simulink model "Reading_Project_model"  (R2019a)
settings: Solver=VariableStepAuto  StartTime=0.0  StopTime=500  MaxStep=0.01  RelTol=1e-3
model workspace: external: MAT-File C:\Kisisel\MATLAB_Workspace\CMP684\NeuralNetworkProject\Lu2018_retry\Lu2018_ws.mat (data not in the file)
values from neighbouring files (symbols this model uses):
  chi = 25    [Reading_Project.mat]    (also in Reading_Project_script.m)
  coupling_matrix = [6.45637  1.27814  2.15629; -1.25619  0.91756  -1.67264; 1.11687  2.48901  -0.83674; 1.23637  -2.6581  -1.12503]    [Reading_Project.mat]    (also in Reading_Project_script.m = [     6.45637     1.27814     2.15629)
  Delta_J = [0  0  0; 0  0  0; 0  0  0]    [Reading_Project.mat]    (also in Reading_Project_script.m = diag([0 0 0]'))
  epsilon = 0.1    [Reading_Project.mat]    (also in Reading_Project_script.m)
  eta_init = [0.01242 0.01584 -0.01749 0.01125]    [Reading_Project.mat]    (also in Reading_Project_script.m = [0.01242, 0.01584, -0.01749, 0.01125]')
  gamma = 0.35    [Reading_Project.mat]    (also in Reading_Project_script.m)
  iota1 = 3    [Reading_Project.mat]    (also in Reading_Project_script.m)
  iota2 = 5    [Reading_Project.mat]    (also in Reading_Project_script.m)
  J = [800.027  0  0; 0  839.93  0; 0  0  289.93]    [Reading_Project.mat]    (also in Reading_Project_script.m = J0 + Delta_J)
  J0 = [800.027  0  0; 0  839.93  0; 0  0  289.93]    [Reading_Project.mat]    (also in Reading_Project_script.m = [  800.027   0           0)
  K = [1.20406729 0 0 0 0 1.62843121 0 0 0 0 2.73505444 0 ... (16 elements, 4x4)]    [Reading_Project.mat]    (also in Reading_Project_script.m = diag(omega_n.^2))
  K1 = [0.5  0  0; 0  0.5  0; 0  0  0.5]    [Reading_Project.mat]    (also in Reading_Project_script.m = diag(k1))
  k1 = [0.5 0.5 0.5]    [Reading_Project.mat]    (also in Reading_Project_script.m = [k11, k12, k13]')
  K2 = [0.5  0  0; 0  0.5  0; 0  0  0.5]    [Reading_Project.mat]    (also in Reading_Project_script.m = diag(k2))
  k2 = [0.5 0.5 0.5]    [Reading_Project.mat]    (also in Reading_Project_script.m = [k21, k22, k23]')
  L = [0.10973 0 0 0 0 0.153132 0 0 0 0 0.264608 0 ... (16 elements, 4x4)]    [Reading_Project.mat]    (also in Reading_Project_script.m = diag(2*omega_n.*zeta))
  lambda = 0.6    [Reading_Project.mat]    (also in Reading_Project_script.m)
  omega_init = [0 0 0]    [Reading_Project.mat]    (also in Reading_Project_script.m = [0, 0, 0]')
  q_init = [0.3 -0.2 -0.3 0.8832]    [Reading_Project.mat]    (also in Reading_Project_script.m = [0.3, -0.2, -0.3, 0.8832]')
  q_p = 0.6    [Reading_Project.mat]    (also in Reading_Project_script.m)
  qd_init = [0 0 0 1]    [Reading_Project.mat]    (also in Reading_Project_script.m = [0, 0, 0, 1]')
  sigma1 = 100    [Reading_Project.mat]    (also in Reading_Project_script.m)
  sigma2 = 0.01    [Reading_Project.mat]    (also in Reading_Project_script.m)
  tau = 10    [Reading_Project.mat]    (also in Reading_Project_script.m)
  um = 68    [Reading_Project.mat]    (also in Reading_Project_script.m)
  weight_init = [0.814723686393 0.905791937076 0.126986816294 0.913375856139 0.632359246225 0.0975404049994 0.278498218867 0.546881519205 0.957506835434 0.964888535199 0.157613081678 0.970592781761 ... (75 elements, 3x25)]    [Reading_Project.mat]    (also in Reading_Project_script.m = rand(3,25))
settings Model: Creator=kocab  LastModifiedBy=kocab

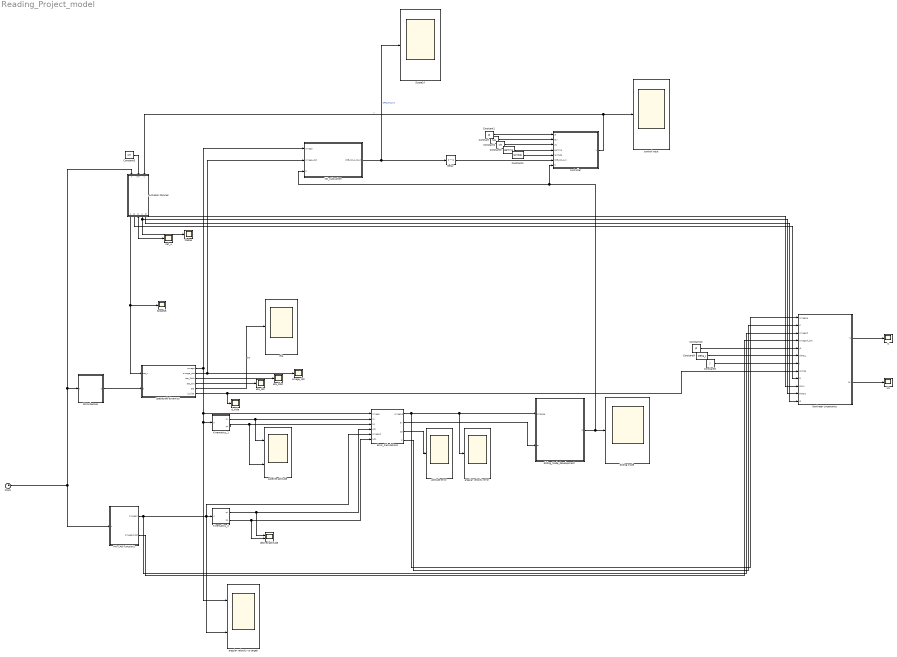
== system Reading_Project_model ==
  Actuator Failures : MATLAB Function  TreatAsAtomicUnit=on
  Clock : Clock
  Constant : Constant  Value=tau
  Constant1 : Constant  Value=J0
  Constant10 : Constant  Value=J0
  Constant2 : Constant  Value=chi
  Constant3 : Constant  Value=gamma
  Constant4 : Constant  Value=lambda
  Constant5 : Constant  Value=um
  Constant8 : Constant  Value=J
  Constant9 : Constant  Value=Delta_J
  Delay : Delay  DelayLength=1  InitialCondition=zeros(3,1)
  Disturbances : MATLAB Function  TreatAsAtomicUnit=on
  Error_Calculations : Subsystem
  Kinematics_1 : Subsystem
  Kinematics_2 : Subsystem
  MATLAB Function1 : MATLAB Function  TreatAsAtomicUnit=on
  N : Scope
  N1 : Scope
  NN_subsystem : Subsystem
  Nonlinear Uncertainty : MATLAB Function  TreatAsAtomicUnit=on
  Scope14 : Scope
  Scope15 : Scope
  Sliding mode : Scope
  Sliding_Mode_Development : Subsystem
  Spacecraft dynamics : Subsystem
  angular velocity error : Scope
  angular velocity vs target : Scope  NumInputPorts=2
  attitude error : Scope
  control input : Scope
  controller : MATLAB Function  TreatAsAtomicUnit=on
  d_tilda : Scope
  desired attitude : Scope  NumInputPorts=2
  eta : Scope
  eta_2dot : Scope
  eta_dot : Scope
  omega_dot : Scope
  sat_u : Scope
  satellite attitude : Scope  NumInputPorts=2
  thetao : Scope
  wires:
  Spacecraft dynamics/1(omega) -> angular velocity vs target/1, Kinematics_1/1(w), Error_Calculations/1(omega), NN_subsystem/1(omega)
  Spacecraft dynamics/5(eta) -> eta/1  "eta"
  Spacecraft dynamics/4(eta_dot) -> eta_dot/1
  Spacecraft dynamics/3(eta_2dot) -> eta_2dot/1
  Spacecraft dynamics/2(omega_dot) -> NN_subsystem/2(omega_dot), omega_dot/1
  MATLAB Function1/1(omegad) -> angular velocity vs target/2, Kinematics_2/1(w), Error_Calculations/5(omegad), Nonlinear Uncertainty/3(omegad)
  Clock/1 -> Actuator Failures/1(t), Disturbances/1(t), MATLAB Function1/1(t)
  Kinematics_1/1(qv) -> satellite attitude/1, Error_Calculations/2(qv)
  Kinematics_1/2(q4) -> satellite attitude/2, Error_Calculations/3(q4)
  Kinematics_2/2(q4) -> desired attitude/2, Error_Calculations/6(qd4)
  Kinematics_2/1(qv) -> Error_Calculations/4(qdv), desired attitude/1
  Disturbances/1(d) -> Spacecraft dynamics/2(d)
  Sliding_Mode_Development/1(S) -> NN_subsystem/3(S), controller/7(S), Sliding mode/1
  NN_subsystem/1(CPB_NN_output) -> Scope14/1, Delay/1  "CPB_NN_out"
  Constant/1 -> controller/2(tau)
  Constant1/1 -> controller/1(J0)
  Constant2/1 -> controller/3(chi)
  Constant3/1 -> controller/4(gamma)
  Constant4/1 -> controller/5(lambda)
  Error_Calculations/1(omegae) -> angular velocity error/1, Sliding_Mode_Development/1(omegae), Nonlinear Uncertainty/1(omegae)
  Error_Calculations/2(ev) -> Sliding_Mode_Development/2(ev)
  Error_Calculations/3(qe) -> attitude error/1
  Actuator Failures/4(thetao) -> thetao/1, Nonlinear Uncertainty/11(thetao)
  Actuator Failures/2(D) -> Nonlinear Uncertainty/9(D)
  Constant8/1 -> Nonlinear Uncertainty/7(J)
  Constant9/1 -> Nonlinear Uncertainty/6(delta_J)
  Constant10/1 -> Nonlinear Uncertainty/5(J0)
  Error_Calculations/4(C) -> Nonlinear Uncertainty/2(C)
  MATLAB Function1/2(omegad_dot) -> Nonlinear Uncertainty/4(omegad_dot)
  Spacecraft dynamics/6(d_tilda) -> Nonlinear Uncertainty/8(d_tilda), d_tilda/1
  Nonlinear Uncertainty/1(N) -> N/1
  controller/1(u) -> Actuator Failures/3(u), control input/1  "u"
  Delay/1 -> controller/6(CPB_NN_out)
  Nonlinear Uncertainty/2(N1) -> N1/1
  Actuator Failures/1(real_torque) -> Scope15/1, Spacecraft dynamics/1(sat_u)
  Constant5/1 -> Actuator Failures/2(um)
  Actuator Failures/3(sat_u) -> sat_u/1, Nonlinear Uncertainty/10(sat_u)
  Actuator Failures/5(G) -> Nonlinear Uncertainty/12(G)

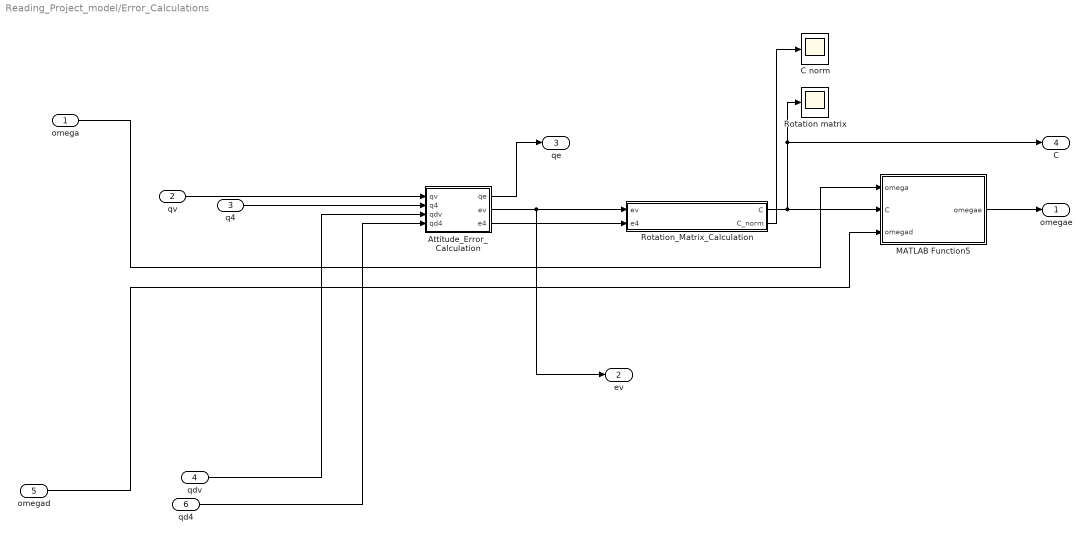
== system Reading_Project_model/Error_Calculations ==
  omega : Inport
  qv : Inport  Port=2
  q4 : Inport  Port=3
  qdv : Inport  Port=4
  omegad : Inport  Port=5
  qd4 : Inport  Port=6
  Attitude_Error_Calculation : MATLAB Function  TreatAsAtomicUnit=on
  C norm : Scope
  MATLAB Function5 : MATLAB Function  TreatAsAtomicUnit=on
  Rotation matrix : Scope
  Rotation_Matrix_Calculation : MATLAB Function  TreatAsAtomicUnit=on
  omegae : Outport
  ev : Outport  Port=2
  qe : Outport  Port=3
  C : Outport  Port=4
  wires:
  q4/1 -> Attitude_Error_Calculation/2(q4)
  Rotation_Matrix_Calculation/1(C) -> C/1, Rotation matrix/1, MATLAB Function5/2(C)
  Rotation_Matrix_Calculation/2(C_norm) -> C norm/1
  omega/1 -> MATLAB Function5/1(omega)
  Attitude_Error_Calculation/2(ev) -> ev/1, Rotation_Matrix_Calculation/1(ev)
  qdv/1 -> Attitude_Error_Calculation/3(qdv)
  Attitude_Error_Calculation/3(e4) -> Rotation_Matrix_Calculation/2(e4)
  qv/1 -> Attitude_Error_Calculation/1(qv)
  qd4/1 -> Attitude_Error_Calculation/4(qd4)
  MATLAB Function5/1(omegae) -> omegae/1
  Attitude_Error_Calculation/1(qe) -> qe/1
  omegad/1 -> MATLAB Function5/3(omegad)

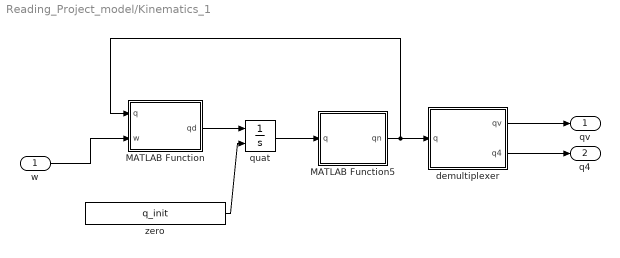
== system Reading_Project_model/Kinematics_1 ==
  w : Inport
  MATLAB Function : MATLAB Function  TreatAsAtomicUnit=on
  MATLAB Function5 : MATLAB Function  TreatAsAtomicUnit=on
  demultiplexer : MATLAB Function  TreatAsAtomicUnit=on
  quat : Integrator  InitialConditionSource=external
  zero : Constant  Value=q_init
  qv : Outport  VectorParamsAs1DForOutWhenUnconnected=on
  q4 : Outport  Port=2  VectorParamsAs1DForOutWhenUnconnected=on
  wires:
  quat/1 -> MATLAB Function5/1(q)
  zero/1 -> quat/2
  MATLAB Function/1(qd) -> quat/1
  w/1 -> MATLAB Function/2(w)
  MATLAB Function5/1(qn) -> demultiplexer/1(q), MATLAB Function/1(q)
  demultiplexer/1(qv) -> qv/1
  demultiplexer/2(q4) -> q4/1

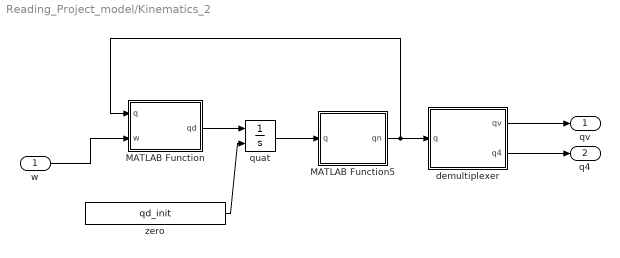
== system Reading_Project_model/Kinematics_2 ==
  w : Inport
  MATLAB Function : MATLAB Function  TreatAsAtomicUnit=on
  MATLAB Function5 : MATLAB Function  TreatAsAtomicUnit=on
  demultiplexer : MATLAB Function  TreatAsAtomicUnit=on
  quat : Integrator  InitialConditionSource=external
  zero : Constant  Value=qd_init
  qv : Outport  VectorParamsAs1DForOutWhenUnconnected=on
  q4 : Outport  Port=2  VectorParamsAs1DForOutWhenUnconnected=on
  wires:
  quat/1 -> MATLAB Function5/1(q)
  zero/1 -> quat/2
  MATLAB Function/1(qd) -> quat/1
  w/1 -> MATLAB Function/2(w)
  MATLAB Function5/1(qn) -> demultiplexer/1(q), MATLAB Function/1(q)
  demultiplexer/1(qv) -> qv/1
  demultiplexer/2(q4) -> q4/1

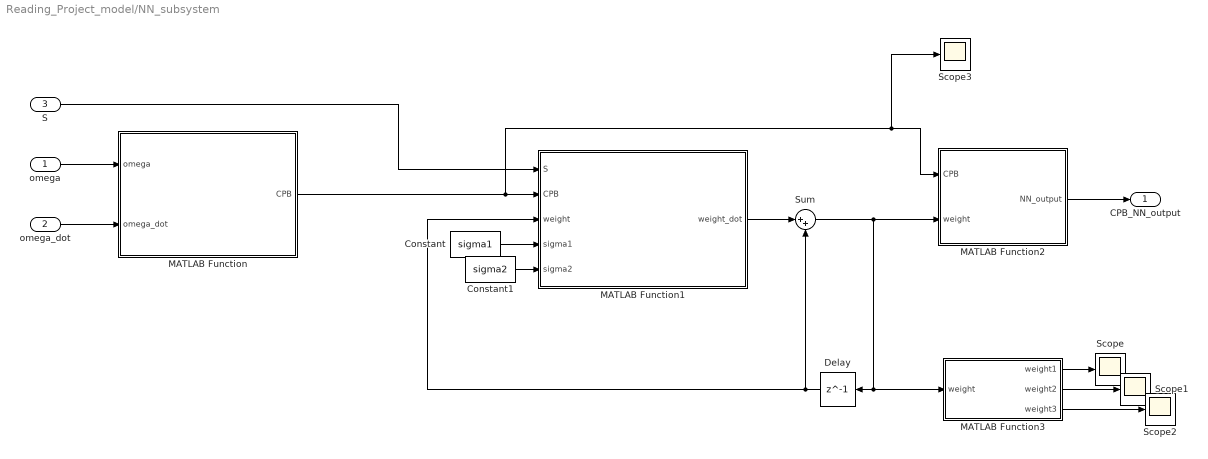
== system Reading_Project_model/NN_subsystem ==
  omega : Inport
  omega_dot : Inport  Port=2
  S : Inport  Port=3
  Constant : Constant  Value=sigma1
  Constant1 : Constant  Value=sigma2
  Delay : Delay  DelayLength=1  InitialCondition=weight_init
  MATLAB Function : MATLAB Function  TreatAsAtomicUnit=on
  MATLAB Function1 : MATLAB Function  TreatAsAtomicUnit=on
  MATLAB Function2 : MATLAB Function  TreatAsAtomicUnit=on
  MATLAB Function3 : MATLAB Function  TreatAsAtomicUnit=on
  Scope{,1..3} (4 alike) : Scope
  Sum : Sum  Inputs=|++
  CPB_NN_output : Outport
  wires:
  omega/1 -> MATLAB Function/1(omega)
  omega_dot/1 -> MATLAB Function/2(omega_dot)
  MATLAB Function/1(CPB) -> Scope3/1, MATLAB Function2/1(CPB), MATLAB Function1/2(CPB)
  S/1 -> MATLAB Function1/1(S)
  Constant/1 -> MATLAB Function1/4(sigma1)
  Constant1/1 -> MATLAB Function1/5(sigma2)
  MATLAB Function2/1(NN_output) -> CPB_NN_output/1
  MATLAB Function3/1(weight1) -> Scope/1
  MATLAB Function3/2(weight2) -> Scope1/1
  MATLAB Function3/3(weight3) -> Scope2/1
  Sum/1 -> MATLAB Function3/1(weight), Delay/1, MATLAB Function2/2(weight)
  Delay/1 -> MATLAB Function1/3(weight), Sum/2
  MATLAB Function1/1(weight_dot) -> Sum/1

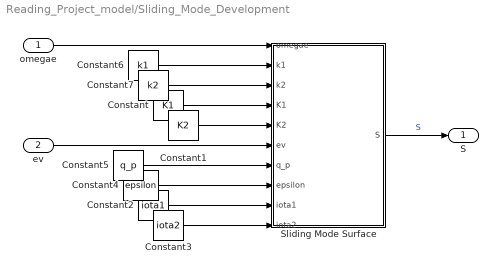
== system Reading_Project_model/Sliding_Mode_Development ==
  omegae : Inport
  ev : Inport  Port=2
  Constant : Constant  Value=K1
  Constant1 : Constant  Value=K2
  Constant2 : Constant  Value=iota1
  Constant3 : Constant  Value=iota2
  Constant4 : Constant  Value=epsilon
  Constant5 : Constant  Value=q_p
  Constant6 : Constant  Value=k1
  Constant7 : Constant  Value=k2
  Sliding Mode Surface : MATLAB Function  TreatAsAtomicUnit=on
  S : Outport
  wires:
  Constant6/1 -> Sliding Mode Surface/2(k1)
  Constant2/1 -> Sliding Mode Surface/9(iota1)
  Constant3/1 -> Sliding Mode Surface/10(iota2)
  Constant7/1 -> Sliding Mode Surface/3(k2)
  Sliding Mode Surface/1(S) -> S/1  "S"
  Constant5/1 -> Sliding Mode Surface/7(q_p)
  Constant/1 -> Sliding Mode Surface/4(K1)
  Constant4/1 -> Sliding Mode Surface/8(epsilon)
  Constant1/1 -> Sliding Mode Surface/5(K2)
  ev/1 -> Sliding Mode Surface/6(ev)
  omegae/1 -> Sliding Mode Surface/1(omegae)

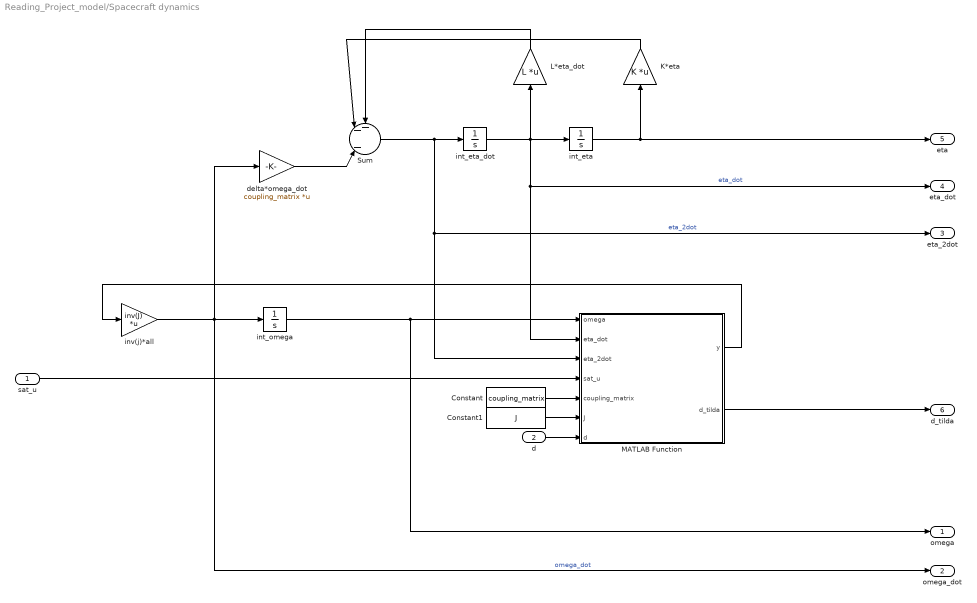
== system Reading_Project_model/Spacecraft dynamics ==
  sat_u : Inport
  d : Inport  Port=2
  Constant : Constant  Value=coupling_matrix
  Constant1 : Constant  Value=J
  K*eta : Gain  Gain=K  Multiplication=Matrix(K*u)
  L*eta_dot : Gain  Gain=L  Multiplication=Matrix(K*u)
  MATLAB Function : MATLAB Function  TreatAsAtomicUnit=on
  Sum : Sum  Inputs=--|-|
  delta*omega_dot : Gain  Gain=coupling_matrix  Multiplication=Matrix(K*u)
  int_eta : Integrator  InitialCondition=eta_init
  int_eta_dot : Integrator  InitialCondition=zeros(4,1)
  int_omega : Integrator  InitialCondition=omega_init
  inv(j)*all : Gain  Gain=inv(J)  Multiplication=Matrix(K*u)
  omega : Outport
  omega_dot : Outport  Port=2
  eta_2dot : Outport  Port=3
  eta_dot : Outport  Port=4
  eta : Outport  Port=5
  d_tilda : Outport  Port=6
  wires:
  int_eta_dot/1 -> MATLAB Function/2(eta_dot), eta_dot/1, L*eta_dot/1, int_eta/1  "eta_dot"
  inv(j)*all/1 -> delta*omega_dot/1, int_omega/1, omega_dot/1  "omega_dot"
  int_eta/1 -> eta/1, K*eta/1
  L*eta_dot/1 -> Sum/1
  K*eta/1 -> Sum/2
  delta*omega_dot/1 -> Sum/3
  Sum/1 -> int_eta_dot/1, eta_2dot/1, MATLAB Function/3(eta_2dot)  "eta_2dot"
  int_omega/1 -> MATLAB Function/1(omega), omega/1
  sat_u/1 -> MATLAB Function/4(sat_u)
  Constant/1 -> MATLAB Function/5(coupling_matrix)
  Constant1/1 -> MATLAB Function/6(J)
  d/1 -> MATLAB Function/7(d)
  MATLAB Function/2(d_tilda) -> d_tilda/1
  MATLAB Function/1(y) -> inv(j)*all/1

== matlab function Reading_Project_model/Spacecraft dynamics/MATLAB Function ==
  data: omega input; eta_dot input; eta_2dot input; sat_u input; coupling_matrix input; J input; y output; d_tilda output; d input
function [y, d_tilda] = fcn(omega, eta_dot, eta_2dot, sat_u, coupling_matrix, J, d)
temp1 =     [0  -omega(3)   omega(2);
            omega(3)    0   -omega(1);
            -omega(2)   omega(1)    0];
        
y = sat_u ...
    - coupling_matrix'*eta_2dot ...
    - temp1 * (J * omega + coupling_matrix' * eta_dot)...
    + d ;

d_tilda = d ...
          - coupling_matrix' * eta_2dot ...
          - temp1 * coupling_matrix' * eta_dot;

== matlab function Reading_Project_model/Kinematics_1/MATLAB Function ==
  data: q input; qd output; w input
function qd = quat(q,w)
%Kinematics
qd = hat4(w)*q/2;

== matlab function Reading_Project_model/Kinematics_1/MATLAB Function5 ==
  data: q input; qn output
function qn = normalize(q)
%quaternion normalization
qn = q/sqrt(sum(q.^2));

== matlab function Reading_Project_model/MATLAB Function1 ==
  data: t input; omegad output; omegad_dot output
function [omegad, omegad_dot] = desired_ang_vel(t)

omegad = 0.05 * [sin(pi*t/100), sin(2*pi*t/100), sin(3*pi*t/100)]';
omegad_dot = 0.05 * (pi/100) * [cos(pi*t/100), 2*cos(2*pi*t/100), 3*cos(3*pi*t/100)]';

== matlab function Reading_Project_model/Error_Calculations/Attitude_Error_Calculation ==
  data: qv input; qe output; q4 input; qdv input; qd4 input; ev output; e4 output
function [qe, ev, e4] = fcn(qv, q4, qdv, qd4)

temp1 =     [0      -qdv(3)   qdv(2);
            qdv(3)    0      -qdv(1);
            -qdv(2)   qdv(1)    0];

% equation 10
ev =    qd4 * qv ...
        - temp1 * qv...
        - q4 * qdv   ;

% equation 11
e4 =    qdv' * qv ...
        + q4 * qd4   ;
    
qe = [ev ; e4];

== matlab function Reading_Project_model/Error_Calculations/Rotation_Matrix_Calculation ==
  data: ev input; e4 input; C output; C_norm output
function [C, C_norm] = rotation_matrix(ev, e4)

temp1 =     [0      -ev(3)   ev(2);
            ev(3)    0      -ev(1);
            -ev(2)   ev(1)    0];

C = (e4^2 - ev' * ev) * eye(3) ...
    + 2 * (ev * ev') ...
    - 2 * e4 * temp1 ;

C_norm = norm(C);

== matlab function Reading_Project_model/Kinematics_2/MATLAB Function ==
  data: q input; qd output; w input
function qd = quat(q,w)
%Kinematics
qd = hat4(w)*q/2;

== matlab function Reading_Project_model/Kinematics_2/MATLAB Function5 ==
  data: q input; qn output
function qn = normalize(q)
%quaternion normalization
qn = q/sqrt(sum(q.^2));

== matlab function Reading_Project_model/Kinematics_2/demultiplexer ==
  data: q input; qv output; q4 output
function [qv, q4] = fcn(q)

qv = q(1:3) ;
q4 = q(4) ;

== matlab function Reading_Project_model/Kinematics_1/demultiplexer ==
  data: q input; qv output; q4 output
function [qv, q4] = fcn(q)

qv = q(1:3) ;
q4 = q(4) ;

== matlab function Reading_Project_model/Disturbances ==
  data: t input; d output
function d = disturbances(t)

%d = [10 * sin(0.1*t), 15 * sin(0.2*t), 20 * sin(0.2*t)]';
d = zeros(3,1);

== matlab function Reading_Project_model/Sliding_Mode_Development/Sliding Mode Surface ==
  data: omegae input; k1 input; k2 input; S output; K1 input; K2 input; ev input; q_p input; epsilon input; iota1 input; iota2 input
function S = sliding_mode(omegae, k1, k2, K1, K2, ev ,q_p, epsilon, iota1, iota2)
Sc = zeros(3,1) ;
temp1 = sign(ev) .* abs(ev).^q_p ; % ei^(q/p)
Si_line =   omegae ...
            + k1 .* ev ...
            + k2 .* temp1 ;

% Calculate Sc (3x1)
for i=1:3
    if Si_line(i) ~= 0
        if abs(ev(i)) >= epsilon
            Sc(i) = temp1(i) ;
        else
            Sc(i) = iota1 * ev(i) ...
                    + iota2 * sign(ev(i)) * ((ev(i))^2) ;
        end
    else
        Sc(i) = temp1(i) ;
    end
end

S = omegae ...
    + K1 * ev ...
    + K2 * Sc ;

== matlab function Reading_Project_model/Error_Calculations/MATLAB Function5 ==
  data: omega input; omegae output; C input; omegad input
function omegae = rel_ang_vel(omega, C, omegad)

omegae = omega - C * omegad ;

== matlab function Reading_Project_model/controller ==
  data: J0 input; tau input; chi input; gamma input; lambda input; CPB_NN_out input; S input; u output
function u   = controller(J0, tau, chi, gamma, lambda, CPB_NN_out, S)
% constants : J0, tau, chi, gamma, lambda
% inputs    : S, WZeta
    
% Actuator control vector
u           = J0 * (- (tau+1/chi) * S...
                    - gamma * (abs(S).^lambda.*sign(S))...
                    - CPB_NN_out...
                    ) ;

== matlab function Reading_Project_model/NN_subsystem/MATLAB Function3 ==
  data: weight input; weight1 output; weight2 output; weight3 output
function [weight1, weight2, weight3] = fcn(weight)

weight1 = weight(1,:);
weight2 = weight(2,:);
weight3 = weight(3,:);

== matlab function Reading_Project_model/Nonlinear Uncertainty ==
  data: N output; omegae input; N1 output; C input; omegad input; omegad_dot input; J0 input; delta_J input; J input; d_tilda input; D input; sat_u input; thetao input; G input
function [N, N1] = nonlinear_uncertainty(omegae, C, omegad, omegad_dot, J0, delta_J, J, d_tilda, D, sat_u, thetao, G)
% omegae+C*Omegad
temp1 = omegae + C * omegad ;
% skew_matrix of (omegae+C*Omegad)
temp2 = [0, -temp1(3), temp1(2);
         temp1(3), 0, -temp1(1);
         -temp1(2), temp1(1), 0];
% skew_matrix of omegae
temp3 = [0, -omegae(3), omegae(2);
         omegae(3), 0, -omegae(1);
         -omegae(2), omegae(1), 0];
     
% N, N1 initialization
N  = zeros(3,1);
N1 = zeros(3,1);
     
     
% equation 24     
N =     - temp2 * delta_J * temp1 ...
        + (eye(3) - delta_J * inv(J)) * d_tilda ...
        + delta_J * (temp3 * C * omegad - C * omegad_dot) ...
        - delta_J * inv(J) * J * (temp3 * C * omegad - C * omegad_dot) ...
        + delta_J * inv(J) * temp2 * J * temp1 ...
        + D * thetao ...
        - delta_J * inv(J) * D * sat_u ...
        + (eye(3) - delta_J * inv(J)) * G ;
    

N1 =    inv(J0) * N ;

== matlab function Reading_Project_model/NN_subsystem/MATLAB Function ==
  data: omega input; CPB output; omega_dot input
function CPB = ChebyshevPolynomials(omega, omega_dot)
CPB = zeros(25,1) ;
CPB =   [   1 ;

            omega(1) ; 
            2*omega(1)^2 - 1 ;
            4*omega(1)^3 - 3*omega(1) ;
            8*omega(1)^4 - 8*omega(1)^2 + 1 ;
            
            omega(2) ; 
            2*omega(2)^2 - 1 ;
            4*omega(2)^3 - 3*omega(2) ;
            8*omega(2)^4 - 8*omega(2)^2 + 1 ;
            
            omega(3) ; 
            2*omega(3)^2 - 1 ;
            4*omega(3)^3 - 3*omega(3) ;
            8*omega(3)^4 - 8*omega(3)^2 + 1 ;
            
            omega_dot(1) ; 
            2*omega_dot(1)^2 - 1 ;
            4*omega_dot(1)^3 - 3*omega_dot(1) ;
            8*omega_dot(1)^4 - 8*omega_dot(1)^2 + 1 ;
            
            omega_dot(2) ; 
            2*omega_dot(2)^2 - 1 ;
            4*omega_dot(2)^3 - 3*omega_dot(2) ;
            8*omega_dot(2)^4 - 8*omega_dot(2)^2 + 1 ;
            
            omega_dot(3) ; 
            2*omega_dot(3)^2 - 1 ;
            4*omega_dot(3)^3 - 3*omega_dot(3) ;
            8*omega_dot(3)^4 - 8*omega_dot(3)^2 + 1 ;
        ] ;

== matlab function Reading_Project_model/NN_subsystem/MATLAB Function1 ==
  settings: updateMethod=DISCRETE
  data: S input; CPB input; weight_dot output; weight input; sigma1 input; sigma2 input
function weight_dot = weight_update(S, CPB, weight, sigma1, sigma2)
weight_dot = rand(3,25) ;
weight_dot =    sigma1 * (S * CPB') ...
                - sigma1 * sigma2 * weight ;

== matlab function Reading_Project_model/NN_subsystem/MATLAB Function2 ==
  data: CPB input; NN_output output; weight input
function NN_output = CPB_NN(CPB, weight)

NN_output = weight * CPB;
% NN_output = zeros(3,1);

== matlab function Reading_Project_model/Actuator Failures ==
  data: real_torque output; D output; sat_u output; thetao output; t input; um input; G output; u input
function [real_torque, D, sat_u, thetao, G] = Actuator_failures(t, um, u)
    % Actuator fault assumptions eq(51) and eq(52)
    if t<15 %15
        G = zeros(3,1);
    else
        G = (0.5+0.25*sin(0.2*t+pi/4))*ones(3,1);
    end
    if t<10  %10
        delta_o     = ones(3,1);
    else
        delta_o     = (0.75+0.1*sin(0.5*t+pi/3))*ones(3,1);
    end
    D       =   diag(delta_o);
    
    thetao = zeros(3,1) ;
    % equation 5
    for i=1:3
        if abs(u(i)) > um
            thetao(i) = sign(u(i)) * um - u(i);
        else
            thetao(i) = 0;
        end
    end
    sat_u = thetao + u;
    real_torque = D * sat_u + G;
